simulink model "example3"  (Simulink 7.1)
settings: Solver=ode45  StartTime=0.0  StopTime=20  MaxStep=0.02  RelTol=1e-4
undefined symbols (not defined in the file): HD, vee
libraries: simulink x1
settings Model: Creator=roy  LastModifiedBy=roy
settings DataIOCC: LimitDataPoints=off

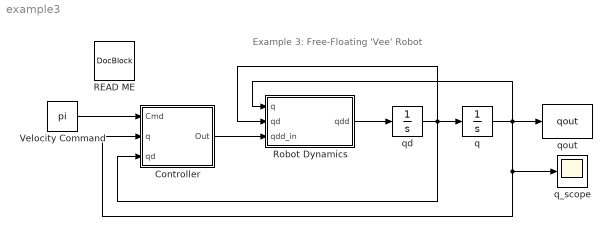
== system example3 ==
  note: Example 3: Free-Floating 'Vee' Robot
  Controller : Subsystem
  READ ME : simulink/Model-Wide Utilities/DocBlock  SystemSampleTime=-1  DocumentType=Text
      content=|
      | This example shows how to simulate a system with a floating base.  In
      | particular, it demonstrates the motion of a simple free-floating mechanism
      | called 'vee', which consists of two rod-shaped bodies connected by a
      | revolute joint.  This mechanism therefore has a total of 7 DoF: six
      | freedoms of overall position and orientation, plus the motion of the
      | revolute joint.  The easiest way to see these freedoms is to run
      | showmotion with the command "showmotion(vee)".  As the time and position
      | data arguments are missing, showmotion gives you a default animation in
      | which each joint is ramped from 0 to 1 and back again.  If you play this
      | default animation, then you will see that the first three freedoms are
      | translations in the X, Y and Z directions, the next three are rotations
      | about the X, Y and Z axes, and the last is the revolute joint connecting
      | the two rods.  The brown lines are not part of the mechanism.  They are
      | just visual guides drawn in fixed locations in space to help you
      | understand the motion.  One line marks the X axis, another the Y axis, a
      | third is at 45 degrees between them, and a fourth joins the centres of
      | mass of the two rods, which are marked with small red spheres.
      |
      | In the simulation, this mechanism floats in a zero-gravity environment,
      | and a simple control system makes the revolute joint turn at a constant
      | rate.  The simulation then shows you how the mechanism as a whole moves in
      | response to the rotation of this joint.
      |
      | The simulation is ready to go: just select 'start', and watch the signals
      | on the scope.  The scope doesn't have a key, so here's a quick summary:
      | the yellow line shooting up is the driven revolute joint (joint 7); the
      | wiggly red line shooting down is the 'Z rotation' (joint 6); the green and
      | blue lines are the Y and X rotations (joints 5 and 4); the cyan line,
      | which is zero, is the Z translation (joint 3); and the magenta line,
      | together with another yellow line hidden underneath it, show the Y and X
      | translations (joints 2 and 1.)  You can now view the animation with
      | "showmotion(vee,tout,qout)".
      |
      | Tip: before playing the animation, see if you can guess what the motion
      | will be.
      |
      | The main new feature in this example is the use of HD (hybrid dynamics) to
      | calculate the dynamics.  This isn't the only way to do it -- one can use
      | one of the forward dynamics routines instead.  The use of HD in this
      | example allows the control system to specify a desired acceleration for
      | the driven joint, instead of a force, and let the dynamics routine work
      | out the correct force to achieve the desired acceleration.  This is akin
      | to a technique in robotics called Computed Torque Control, in which a
      | control law calculates a desired joint acceleration vector, and an inverse
      | dynamics function is used to translate the acceleration into a joint force
      | vector, which is then sent as a command signal to the force servos
      | controlling the individual joints.
      |
      | If you open the block "robot dynamics", you will see that the Matlab
      | function block inside it contains the call
      |
      | HD(vee(1),[1 1 1 1 1 1 0], u(1:7),u(8:14), [zeros(6,1);u(15)], zeros(7,1))
      |
      | which is equivalent to
      |
      | HD( vee(1), [1 1 1 1 1 1 0], q, qd, [zeros(6,1);qdd_in], zeros(7,1) )
      |
      | There are several new things here.  First, vee takes an argument.
      | Changing this argument will alter the length and mass of the second rod.
      | Next, the argument [1 1 1 1 1 1 0] tells HD that the first six joints are
      | to be treated as 'forward-dynamics joints', meaning that the forces at
      | these joints are given and the task is to calculate the accelerations,
      | while the seventh joint is an 'inverse-dynamics joint', meaning that the
      | acceleration has been given and the task is to work out the force.  The
      | next two arguments are the vectors of joint position and velocity
      | variables; and the final two arguments are the vector of given
      | accelerations and the vector of given forces.  The first six elements of
      | the given-acceleration vector are ignored (because the first six joints
      | are forward-dynamics joints), and the seventh is interpreted as the given
      | acceleration for joint 7 (the controlled joint).  Likewise, the first six
      | elements of the given-force vector are interpreted as the given forces at
      | the first six joints and the seventh element is ignored.  The given forces
      | are all zero because there is no force acting between the fixed base (body
      | 0) and the floating base (body 6).  HD then computes both the complete
      | vector of joint accelerations and the complete vector of joint forces.
      | However, Simulink is expecting only a single return value, so it discards
      | the second return value (which conveniently just happens to be the forces)
      | and keeps the first.
      |
      | Something to try:
      |
      | Using showmotion, zoom in a lot on the far end of one of the two rods, and
      | press 0 (zero) several times.  This toggles between the initial and final
      | positions of the simulation.  Theoretically, they should be the same.
      | However, due to truncation error in the numerical integration process,
      | they are slightly different.  (The maximum step size has been set to 0.02
      | in this simulation, which forces Simulink to perform the integration at a
      | high accuracy.)  Now, this is actually a special case caused by the fact
      | that the two rods are identical.  If we make them different, then the
      | motion no longer follows a closed path.  Try changing the argument of vee
      | in the Matlab function block from 1 to 0.7, and re-run the simulation.  To
      | see the result, you will have to use the command
      | "showmotion(vee(0.7),tout,qout)" (i.e., you have to give vee the same
      | argument as used in the simulation, or showmotion will have the wrong
      | model).  The initial and final positions are now definitely not the same.
  Robot Dynamics : Subsystem
  Velocity Command : Constant  Value=pi  OutDataType=sfix(16)  OutScaling=2^0
  q : Integrator
  q_scope : Scope
      settings: YMin=-2  YMax=2
  qd : Integrator
  qout : ToWorkspace  VariableName=qout  SampleTime=-1  SaveFormat=Array
  wires:
  Robot Dynamics/1(qdd) -> qd/1
  qd/1 -> q/1, Robot Dynamics/2(qd), Controller/3(qd)
  q/1 -> qout/1, Robot Dynamics/1(q), q_scope/1, Controller/2(q)
  Velocity Command/1 -> Controller/1(Cmd)
  Controller/1(Out) -> Robot Dynamics/3(qdd_in)

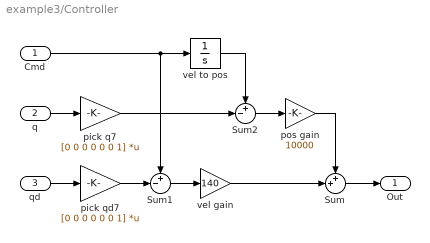
== system example3/Controller ==
  Cmd : Inport  OutDataType=sfix(16)  OutScaling=2^0
  q : Inport  Port=2  OutDataType=sfix(16)  OutScaling=2^0
  qd : Inport  Port=3  OutDataType=sfix(16)  OutScaling=2^0
  Sum : Sum  Inputs=++|  OutDataType=sfix(16)  OutScaling=2^0
  Sum1 : Sum  Inputs=+-|  OutDataType=sfix(16)  OutScaling=2^0
  Sum2 : Sum  Inputs=+-|  OutDataType=sfix(16)  OutScaling=2^0
  pick q7 : Gain  Gain=[0 0 0 0 0 0 1]  Multiplication=Matrix(K*u)  ParameterDataType=sfix(16)  ParameterScaling=2^0  OutDataType=sfix(16)  OutScaling=2^0
  pick qd7 : Gain  Gain=[0 0 0 0 0 0 1]  Multiplication=Matrix(K*u)  ParameterDataType=sfix(16)  ParameterScaling=2^0  OutDataType=sfix(16)  OutScaling=2^0
  pos gain : Gain  Gain=10000  ParameterDataType=sfix(16)  ParameterScaling=2^0  OutDataType=sfix(16)  OutScaling=2^0
  vel gain : Gain  Gain=140  ParameterDataType=sfix(16)  ParameterScaling=2^0  OutDataType=sfix(16)  OutScaling=2^0
  vel to pos : Integrator
  Out : Outport  OutDataType=sfix(16)  OutScaling=2^0
  wires:
  Sum/1 -> Out/1
  Cmd/1 -> vel to pos/1, Sum1/1
  q/1 -> pick q7/1
  qd/1 -> pick qd7/1
  pick qd7/1 -> Sum1/2
  pick q7/1 -> Sum2/2
  vel to pos/1 -> Sum2/1
  Sum2/1 -> pos gain/1
  Sum1/1 -> vel gain/1
  vel gain/1 -> Sum/2
  pos gain/1 -> Sum/1

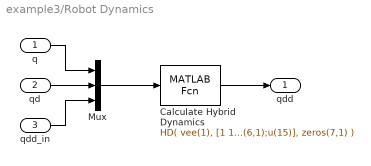
== system example3/Robot Dynamics ==
  q : Inport  OutDataType=sfix(16)  OutScaling=2^0
  qd : Inport  Port=2  OutDataType=sfix(16)  OutScaling=2^0
  qdd_in : Inport  Port=3  OutDataType=sfix(16)  OutScaling=2^0
  Calculate Hybrid Dynamics : MATLABFcn  MATLABFcn=HD( vee(1), [1 1 1 1 1 1 0], u(1:7), u(8:14), [zeros(6,1);u(15)], zeros(7,1) )  OutputDimensions=[7 1]  OutputSignalType=real  Output1D=off
  Mux : Mux  Inputs=3
  qdd : Outport  OutDataType=sfix(16)  OutScaling=2^0
  wires:
  qd/1 -> Mux/2
  q/1 -> Mux/1
  qdd_in/1 -> Mux/3
  Mux/1 -> Calculate Hybrid Dynamics/1
  Calculate Hybrid Dynamics/1 -> qdd/1
